simulink model "lock_srw_vA_mac"  (R2019a)
settings: Solver=VariableStepAuto  StartTime=0.0  StopTime=inf  RelTol=1e-3
undefined symbols (not defined in the file): f
libraries: dspnetwork x9, instrumentlib x9, simulink x2
(part 2 of 2)

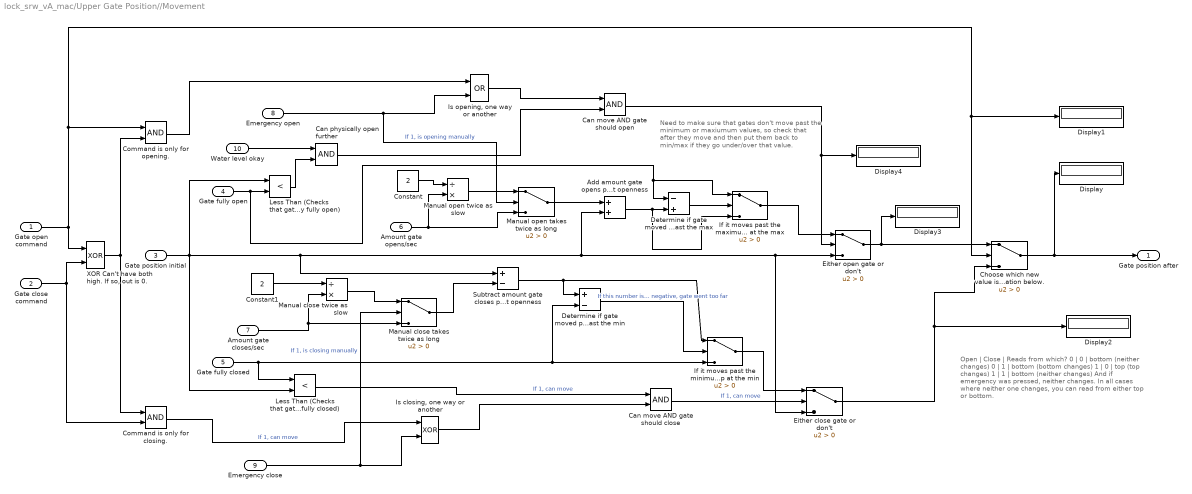
== system lock_srw_vA_mac/Upper Gate Position//Movement ==
  note: Need to make sure that gates don't move past the minimum or maxiumum values, so check that after they move and then put them back to min/max if they go under/over that value.
  note: Open	|	Close	|	Reads from which?
      | 0		|	0		|	bottom (neither changes)
      | 0		|	1		|	bottom (bottom changes)
      | 1		|	0		|	top (top changes)
      | 1		|	1		|	bottom (neither changes)
      |
      | And if emergency was pressed, neither changes.  In all cases where neither one changes, you can read from either top or bottom.
  Gate open command : Inport
  Gate close command : Inport  Port=2
  Gate position initial : Inport  Port=3
  Gate fully open : Inport  Port=4
  Gate fully closed : Inport  Port=5
  Amount gate opens/sec : Inport  Port=6
  Amount gate closes/sec : Inport  Port=7
  Emergency open : Inport  Port=8
  Emergency close : Inport  Port=9
  Water level okay : Inport  Port=10
  Add amount gate opens per second to current openness : Sum
  Can move AND gate should close : Logic  AllPortsSameDT=off  OutDataTypeStr=boolean
  Can move AND gate should open : Logic  AllPortsSameDT=off  OutDataTypeStr=boolean
  Can physically open further : Logic  AllPortsSameDT=off  OutDataTypeStr=boolean
  "Choose which new value is correct, based upon the open command. See annotation below." : Switch  Criteria=u2 > Threshold
  Command is only for closing. : Logic  AllPortsSameDT=off  OutDataTypeStr=boolean
  Command is only for opening. : Logic  AllPortsSameDT=off  OutDataTypeStr=boolean
  Constant : Constant  Value=2
  Constant1 : Constant  Value=2
  Determine if gate moved past the max : Sum  Inputs=-+
  Determine if gate moved past the min : Sum  Inputs=+-
  Display{,1..4} (5 alike) : Display
  Either close gate or don't : Switch  Criteria=u2 > Threshold
  Either open gate or don't : Switch  Criteria=u2 > Threshold
  "If it moves past the maximum, it will stop at the max" : Switch  Criteria=u2 > Threshold
  "If it moves past the minimum, it will stop at the min" : Switch  Criteria=u2 > Threshold
  "Is closing, one way or another" : Logic  Operator=XOR  IconShape=distinctive  AllPortsSameDT=off  OutDataTypeStr=boolean
  "Is opening, one way or another" : Logic  Operator=OR  IconShape=distinctive  AllPortsSameDT=off  OutDataTypeStr=boolean
  Less Than (Checks that gate isn't already fully closed) : RelationalOperator  Operator=<  OutDataTypeStr=boolean  RndMeth=Simplest
  Less Than (Checks that gate isn't already fully open) : RelationalOperator  Operator=<  OutDataTypeStr=boolean  RndMeth=Simplest
  Manual close takes twice as long : Switch  Criteria=u2 > Threshold
  Manual close twice as slow : Product  Inputs=/*
  Manual open takes twice as long : Switch  Criteria=u2 > Threshold
  Manual open twice as slow : Product  Inputs=/*
  Subtract amount gate closes per second from current openness : Sum  Inputs=+-
  "XOR Can't have both high. If so, out is 0." : Logic  Operator=XOR  IconShape=distinctive  AllPortsSameDT=off  OutDataTypeStr=boolean
  Gate position after : Outport
  wires:
  Gate open command/1 -> "Choose which new value is correct, based upon the open command. See annotation below."/2, Display1/1, Command is only for opening./1, "XOR Can't have both high. If so, out is 0."/1
  Gate close command/1 -> Command is only for closing./2, "XOR Can't have both high. If so, out is 0."/2
  "XOR Can't have both high. If so, out is 0."/1 -> Command is only for closing./1, Command is only for opening./2
  Gate position initial/1 -> Less Than (Checks that gate isn't already fully open)/1, Either open gate or don't/3, Either close gate or don't/3, Add amount gate opens per second to current openness/2, Subtract amount gate closes per second from current openness/1, Less Than (Checks that gate isn't already fully closed)/2
  "Choose which new value is correct, based upon the open command. See annotation below."/1 -> Display/1, Gate position after/1
  Can move AND gate should close/1 -> Either close gate or don't/2  "If 1, can move"
  Either open gate or don't/1 -> Display3/1, "Choose which new value is correct, based upon the open command. See annotation below."/1
  Either close gate or don't/1 -> "Choose which new value is correct, based upon the open command. See annotation below."/3, Display2/1
  Less Than (Checks that gate isn't already fully open)/1 -> Can physically open further/2
  Can physically open further/1 -> Can move AND gate should open/2
  Less Than (Checks that gate isn't already fully closed)/1 -> Can move AND gate should close/1  "If 1, can move"
  Water level okay/1 -> Can physically open further/1
  Can move AND gate should open/1 -> Display4/1, Either open gate or don't/2
  Gate fully closed/1 -> "If it moves past the minimum, it will stop at the min"/3, Determine if gate moved past the min/2, Less Than (Checks that gate isn't already fully closed)/1
  "If it moves past the minimum, it will stop at the min"/1 -> Either close gate or don't/1
  Subtract amount gate closes per second from current openness/1 -> Determine if gate moved past the min/1, "If it moves past the minimum, it will stop at the min"/1
  Determine if gate moved past the min/1 -> "If it moves past the minimum, it will stop at the min"/2  "If this number is negative, gate went too far"
  Gate fully open/1 -> "If it moves past the maximum, it will stop at the max"/1, Determine if gate moved past the max/1, Less Than (Checks that gate isn't already fully open)/2
  Determine if gate moved past the max/1 -> "If it moves past the maximum, it will stop at the max"/2
  "If it moves past the maximum, it will stop at the max"/1 -> Either open gate or don't/1
  Add amount gate opens per second to current openness/1 -> Determine if gate moved past the max/2, "If it moves past the maximum, it will stop at the max"/3
  "Is closing, one way or another"/1 -> Can move AND gate should close/2
  Emergency close/1 -> Manual close takes twice as long/2, "Is closing, one way or another"/2  "If 1, is closing manually"
  Command is only for closing./1 -> "Is closing, one way or another"/1  "If 1, can move"
  "Is opening, one way or another"/1 -> Can move AND gate should open/1
  Emergency open/1 -> "Is opening, one way or another"/2, Manual open takes twice as long/2  "If 1, is opening manually"
  Command is only for opening./1 -> "Is opening, one way or another"/1
  Amount gate opens/sec/1 -> Manual open takes twice as long/3, Manual open twice as slow/2
  Manual open twice as slow/1 -> Manual open takes twice as long/1
  Manual open takes twice as long/1 -> Add amount gate opens per second to current openness/1
  Constant/1 -> Manual open twice as slow/1
  Manual close twice as slow/1 -> Manual close takes twice as long/1
  Amount gate closes/sec/1 -> Manual close twice as slow/2, Manual close takes twice as long/3
  Constant1/1 -> Manual close twice as slow/1
  Manual close takes twice as long/1 -> Subtract amount gate closes per second from current openness/2
